simulink model "EiH_VFC_Renew_R2021b"  (R2021b)
settings: Solver=ode4  StartTime=0.0  StopTime=30  FixedStep=0.01  RelTol=1e-3
values from neighbouring files (symbols this model uses):
  denomi_threshold = 1e-8    (= 1e-08)    [param_EiH_VFC.m]
  Keo1 = Keo_Gain    (= 0.5)    [param_EiH_VFC.m]
  Keo2 = Keo_Gain    (= 0.5)    [param_EiH_VFC.m]
  Keo3 = Keo_Gain    (= 0.5)    [param_EiH_VFC.m]
  Keo4 = Keo_Gain    (= 0.5)    [param_EiH_VFC.m]
  Keo5 = Keo_Gain    (= 0.5)    [param_EiH_VFC.m]
  Keo6 = Keo_Gain    (= 0.5)    [param_EiH_VFC.m]
  Km1 = Km_gain    (= 0.1)    [param_EiH_VFC.m]
  Km2 = Km_gain    (= 0.1)    [param_EiH_VFC.m]
  Km3 = Km_gain    (= 0.1)    [param_EiH_VFC.m]
  Km4 = Km_gain    (= 0.1)    [param_EiH_VFC.m]
  Km5 = Km_gain    (= 0.1)    [param_EiH_VFC.m]
  Km6 = Km_gain    (= 0.1)    [param_EiH_VFC.m]
  pco_bar_init = pco_init + [0.15; 0.3; -0.1]    [param_EiH_VFC.m]
  pd = [1.0; 1.0; 0]    [param_EiH_VFC.m]
  Pinho_Para = [0; 0; 0; s_lambda_x; s_lambda_y]    [param_EiH_VFC.m]
  po = [xo1; yo1; zo1; xo2; yo2; zo2; xo3; yo3; zo3; xo4; yo4; zo4]    [param_EiH_VFC.m]
  pzeta_md = [pmd; zetamd]    [param_EiH_VFC.m]
  pzeta_wo_init = [pwo_init;zetawo_init]    [param_EiH_VFC.m]
  qwm_init = [0.0; 0.0; 0.0]    [param_EiH_VFC.m]
  R_threshold = 1e-8    (= 1e-08)    [param_EiH_VFC.m]
  Rco_bar_init = Rfromxi(zetaco_bar_init)    [param_EiH_VFC.m]
  theta_dz = 0.0    (= 0)    [param_EiH_VFC.m]
  zeta_threshold = 1e-8    (= 1e-08)    [param_EiH_VFC.m]
undefined symbols (not defined in the file or in its folder): Angle, Axis, magnitude, sx, sy
libraries: dspnetwork x2, dspmtrx3 x2, robotcorelib x1, vrlib x1
(part 2 of 4)

== system EiH_VFC_Renew_R2021b/make Ad(ge)/wedge ==
  "[3x1]" : Inport
  Product1 : Product  InputSameDT=on  SaturateOnIntegerOverflow=on  OutDataTypeStr=Inherit: Same as first input
  Product2 : Product  InputSameDT=on  SaturateOnIntegerOverflow=on  OutDataTypeStr=Inherit: Same as first input
  Product3 : Product  InputSameDT=on  SaturateOnIntegerOverflow=on  OutDataTypeStr=Inherit: Same as first input
  Sum : Sum  Inputs=+++  InputSameDT=on  SaturateOnIntegerOverflow=on  OutDataTypeStr=Inherit: Same as first input
  Xaxis : Constant  Value=[0 0 0;0 0 -1;0 1 0]  VectorParams1D=off
  Yaxis : Constant  Value=[0 0 1;0 0 0;-1 0 0]  VectorParams1D=off
  Zaxis : Constant  Value=[0 -1 0;1 0 0;0 0 0]  VectorParams1D=off
  x : Gain  Gain=[1 0 0]  Multiplication=Matrix(K*u)  SaturateOnIntegerOverflow=on  OutDataTypeStr=Inherit: Same as input  ParamDataTypeStr=Inherit: Same as input
  y : Gain  Gain=[0 1 0]  Multiplication=Matrix(K*u)  SaturateOnIntegerOverflow=on  OutDataTypeStr=Inherit: Same as input  ParamDataTypeStr=Inherit: Same as input
  z : Gain  Gain=[0 0 1]  Multiplication=Matrix(K*u)  SaturateOnIntegerOverflow=on  OutDataTypeStr=Inherit: Same as input  ParamDataTypeStr=Inherit: Same as input
  "[3x3]" : Outport  VectorParamsAs1DForOutWhenUnconnected=off
  wires:
  Sum/1 -> "[3x3]"/1
  Product1/1 -> Sum/3
  Product2/1 -> Sum/1
  Product3/1 -> Sum/2
  "[3x1]"/1 -> z/1, x/1, y/1
  y/1 -> Product3/1
  Yaxis/1 -> Product3/2
  x/1 -> Product2/1
  Xaxis/1 -> Product2/2
  z/1 -> Product1/1
  Zaxis/1 -> Product1/2

== system EiH_VFC_Renew_R2021b/make Rco pco/make p_zeta co ==
  "pco " : Inport
  Rco : Inport  Port=2
  Data pco : Subsystem
  Data zetaco : Subsystem
  Mux : Mux  Inputs=2
  make zeta_co : Subsystem
  pco WS : Subsystem
  "zeta_co WS " : Subsystem
  tag scope: p_zeta_co=global
  wires:
  "pco "/1 -> Data pco/1("pco "), pco WS/1(pco), Mux/1
  make zeta_co/1(zeta_co) -> "zeta_co WS "/1(zetaco), Data zetaco/1(zetaco), Mux/2
  Mux/1 -> [p_zeta_co]
  Rco/1 -> make zeta_co/1(Rco)

== system EiH_VFC_Renew_R2021b/make Rco pco/wedge ==
  "[3x1]" : Inport
  Product1 : Product  InputSameDT=on  SaturateOnIntegerOverflow=on  OutDataTypeStr=Inherit: Same as first input
  Product2 : Product  InputSameDT=on  SaturateOnIntegerOverflow=on  OutDataTypeStr=Inherit: Same as first input
  Product3 : Product  InputSameDT=on  SaturateOnIntegerOverflow=on  OutDataTypeStr=Inherit: Same as first input
  Sum : Sum  Inputs=+++  InputSameDT=on  SaturateOnIntegerOverflow=on  OutDataTypeStr=Inherit: Same as first input
  Xaxis : Constant  Value=[0 0 0;0 0 -1;0 1 0]  VectorParams1D=off
  Yaxis : Constant  Value=[0 0 1;0 0 0;-1 0 0]  VectorParams1D=off
  Zaxis : Constant  Value=[0 -1 0;1 0 0;0 0 0]  VectorParams1D=off
  x : Gain  Gain=[1 0 0]  Multiplication=Matrix(K*u)  SaturateOnIntegerOverflow=on  OutDataTypeStr=Inherit: Same as input  ParamDataTypeStr=Inherit: Same as input
  y : Gain  Gain=[0 1 0]  Multiplication=Matrix(K*u)  SaturateOnIntegerOverflow=on  OutDataTypeStr=Inherit: Same as input  ParamDataTypeStr=Inherit: Same as input
  z : Gain  Gain=[0 0 1]  Multiplication=Matrix(K*u)  SaturateOnIntegerOverflow=on  OutDataTypeStr=Inherit: Same as input  ParamDataTypeStr=Inherit: Same as input
  "[3x3]" : Outport  VectorParamsAs1DForOutWhenUnconnected=off
  wires:
  Sum/1 -> "[3x3]"/1
  Product1/1 -> Sum/3
  Product2/1 -> Sum/1
  Product3/1 -> Sum/2
  "[3x1]"/1 -> z/1, x/1, y/1
  y/1 -> Product3/1
  Yaxis/1 -> Product3/2
  x/1 -> Product2/1
  Xaxis/1 -> Product2/2
  z/1 -> Product1/1
  Zaxis/1 -> Product1/2

== system EiH_VFC_Renew_R2021b/make Rd pd/make_Rd ==
  zeta_d : Inport
  "3x1 -> 2norm" : Subsystem
  Constant : Constant
  I : Constant  Value=eye(3)  VectorParams1D=off
  I1 : Constant  Value=eye(3)  VectorParams1D=off
  Product : Product  InputSameDT=on  SaturateOnIntegerOverflow=on  OutDataTypeStr=Inherit: Same as first input
  Product1 : Product  InputSameDT=on  SaturateOnIntegerOverflow=on  OutDataTypeStr=Inherit: Same as first input
  Product2 : Product  Inputs=/  InputSameDT=on  SaturateOnIntegerOverflow=on  OutDataTypeStr=Inherit: Same as first input
  Product3 : Product  Multiplication=Matrix(*)  InputSameDT=on  SaturateOnIntegerOverflow=on  OutDataTypeStr=Inherit: Same as first input
  Product4 : Product  InputSameDT=on  SaturateOnIntegerOverflow=on  OutDataTypeStr=Inherit: Same as first input
  Sum : Sum  Inputs=+++  InputSameDT=on  SaturateOnIntegerOverflow=on  OutDataTypeStr=Inherit: Same as first input
  Sum1 : Sum  Inputs=|+-  InputSameDT=on  SaturateOnIntegerOverflow=on  OutDataTypeStr=Inherit: Same as first input
  Switch : Switch  Threshold=R_threshold  SaturateOnIntegerOverflow=on  InputSameDT=on
  cos(theta) : Trigonometry  Operator=cos
  sin(theta) : Trigonometry
  wedge : Subsystem
  zero check R_threshold : Subsystem
  Rd : Outport  VectorParamsAs1DForOutWhenUnconnected=off
  wires:
  Product3/1 -> Product1/1
  zeta_d/1 -> wedge/1("[3x1]"), "3x1 -> 2norm"/1(3x1)
  Product2/1 -> Product/2
  zero check R_threshold/1(Out1) -> cos(theta)/1, Switch/2, sin(theta)/1, Product2/1
  wedge/1("[3x3]") -> Product/1
  Product/1 -> Product3/2, Product3/1, Product4/1
  "3x1 -> 2norm"/1(2 norm) -> zero check R_threshold/1(In1)
  Switch/1 -> Rd/1
  I1/1 -> Switch/3
  Sum/1 -> Switch/1
  sin(theta)/1 -> Product4/2
  I/1 -> Sum/1
  Constant/1 -> Sum1/1
  cos(theta)/1 -> Sum1/2
  Sum1/1 -> Product1/2
  Product1/1 -> Sum/3
  Product4/1 -> Sum/2

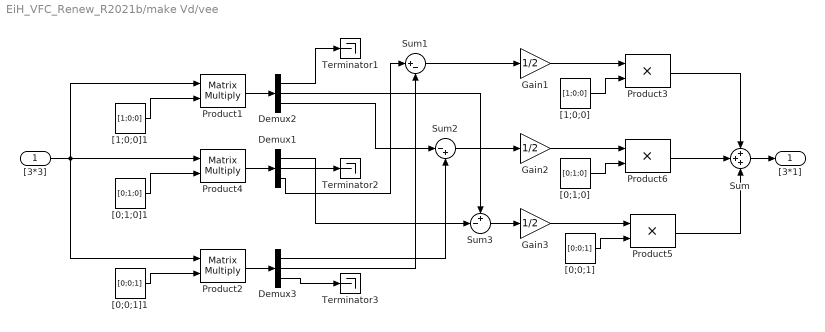
== system EiH_VFC_Renew_R2021b/make Vd/vee ==
  "[3*3]" : Inport
  Demux1 : Demux  Outputs=3
      settings: DisplayOption=none
  Demux2 : Demux  Outputs=3
      settings: DisplayOption=none
  Demux3 : Demux  Outputs=3
      settings: DisplayOption=none
  Gain1 : Gain  Gain=1/2  SaturateOnIntegerOverflow=on  OutDataTypeStr=Inherit: Same as input  ParamDataTypeStr=Inherit: Same as input
  Gain2 : Gain  Gain=1/2  SaturateOnIntegerOverflow=on  OutDataTypeStr=Inherit: Same as input  ParamDataTypeStr=Inherit: Same as input
  Gain3 : Gain  Gain=1/2  SaturateOnIntegerOverflow=on  OutDataTypeStr=Inherit: Same as input  ParamDataTypeStr=Inherit: Same as input
  Product1 : Product  Multiplication=Matrix(*)  InputSameDT=on  SaturateOnIntegerOverflow=on  OutDataTypeStr=Inherit: Same as first input
  Product2 : Product  Multiplication=Matrix(*)  InputSameDT=on  SaturateOnIntegerOverflow=on  OutDataTypeStr=Inherit: Same as first input
  Product3 : Product  InputSameDT=on  SaturateOnIntegerOverflow=on  OutDataTypeStr=Inherit: Same as first input
  Product4 : Product  Multiplication=Matrix(*)  InputSameDT=on  SaturateOnIntegerOverflow=on  OutDataTypeStr=Inherit: Same as first input
  Product5 : Product  InputSameDT=on  SaturateOnIntegerOverflow=on  OutDataTypeStr=Inherit: Same as first input
  Product6 : Product  InputSameDT=on  SaturateOnIntegerOverflow=on  OutDataTypeStr=Inherit: Same as first input
  Sum : Sum  Inputs=+++  InputSameDT=on  SaturateOnIntegerOverflow=on  OutDataTypeStr=Inherit: Same as first input
  Sum1 : Sum  Inputs=|+-  InputSameDT=on  SaturateOnIntegerOverflow=on  OutDataTypeStr=Inherit: Same as first input
  Sum2 : Sum  Inputs=|-+  InputSameDT=on  SaturateOnIntegerOverflow=on  OutDataTypeStr=Inherit: Same as first input
  Sum3 : Sum  Inputs=+-|  InputSameDT=on  SaturateOnIntegerOverflow=on  OutDataTypeStr=Inherit: Same as first input
  Terminator1 : Terminator
  Terminator2 : Terminator
  Terminator3 : Terminator
  "[0;0;1]" : Constant  Value=[0;0;1]  VectorParams1D=off
  "[0;0;1]1" : Constant  Value=[0;0;1]  VectorParams1D=off
  "[0;1;0]" : Constant  Value=[0;1;0]  VectorParams1D=off
  "[0;1;0]1" : Constant  Value=[0;1;0]  VectorParams1D=off
  "[1;0;0]" : Constant  Value=[1;0;0]  VectorParams1D=off
  "[1;0;0]1" : Constant  Value=[1;0;0]  VectorParams1D=off
  "[3*1]" : Outport  VectorParamsAs1DForOutWhenUnconnected=off
  wires:
  Demux1/1 -> Sum3/2
  Demux2/2 -> Sum3/1
  Sum3/1 -> Gain3/1
  Sum2/1 -> Gain2/1
  Demux2/3 -> Sum2/1
  Gain3/1 -> Product5/1
  Gain2/1 -> Product6/1
  Demux3/2 -> Sum1/2
  Gain1/1 -> Product3/1
  Sum1/1 -> Gain1/1
  Sum/1 -> "[3*1]"/1
  Product3/1 -> Sum/1
  Product5/1 -> Sum/3
  Product6/1 -> Sum/2
  "[0;0;1]"/1 -> Product5/2
  "[0;1;0]"/1 -> Product6/2
  "[1;0;0]"/1 -> Product3/2
  Demux3/1 -> Sum2/2
  Demux3/3 -> Terminator3/1
  Product2/1 -> Demux3/1
  "[0;0;1]1"/1 -> Product2/2
  Demux2/1 -> Terminator1/1
  Product1/1 -> Demux2/1
  "[1;0;0]1"/1 -> Product1/2
  Demux1/3 -> Sum1/1
  Demux1/2 -> Terminator2/1
  Product4/1 -> Demux1/1
  "[0;1;0]1"/1 -> Product4/2
  "[3*3]"/1 -> Product1/1, Product2/1, Product4/1

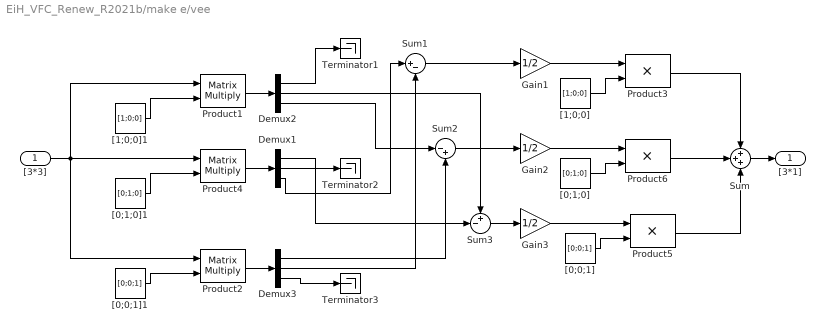
== system EiH_VFC_Renew_R2021b/make e/vee ==
  "[3*3]" : Inport
  Demux1 : Demux  Outputs=3
      settings: DisplayOption=none
  Demux2 : Demux  Outputs=3
      settings: DisplayOption=none
  Demux3 : Demux  Outputs=3
      settings: DisplayOption=none
  Gain1 : Gain  Gain=1/2  SaturateOnIntegerOverflow=on  OutDataTypeStr=Inherit: Same as input  ParamDataTypeStr=Inherit: Same as input
  Gain2 : Gain  Gain=1/2  SaturateOnIntegerOverflow=on  OutDataTypeStr=Inherit: Same as input  ParamDataTypeStr=Inherit: Same as input
  Gain3 : Gain  Gain=1/2  SaturateOnIntegerOverflow=on  OutDataTypeStr=Inherit: Same as input  ParamDataTypeStr=Inherit: Same as input
  Product1 : Product  Multiplication=Matrix(*)  InputSameDT=on  SaturateOnIntegerOverflow=on  OutDataTypeStr=Inherit: Same as first input
  Product2 : Product  Multiplication=Matrix(*)  InputSameDT=on  SaturateOnIntegerOverflow=on  OutDataTypeStr=Inherit: Same as first input
  Product3 : Product  InputSameDT=on  SaturateOnIntegerOverflow=on  OutDataTypeStr=Inherit: Same as first input
  Product4 : Product  Multiplication=Matrix(*)  InputSameDT=on  SaturateOnIntegerOverflow=on  OutDataTypeStr=Inherit: Same as first input
  Product5 : Product  InputSameDT=on  SaturateOnIntegerOverflow=on  OutDataTypeStr=Inherit: Same as first input
  Product6 : Product  InputSameDT=on  SaturateOnIntegerOverflow=on  OutDataTypeStr=Inherit: Same as first input
  Sum : Sum  Inputs=+++  InputSameDT=on  SaturateOnIntegerOverflow=on  OutDataTypeStr=Inherit: Same as first input
  Sum1 : Sum  Inputs=|+-  InputSameDT=on  SaturateOnIntegerOverflow=on  OutDataTypeStr=Inherit: Same as first input
  Sum2 : Sum  Inputs=|-+  InputSameDT=on  SaturateOnIntegerOverflow=on  OutDataTypeStr=Inherit: Same as first input
  Sum3 : Sum  Inputs=+-|  InputSameDT=on  SaturateOnIntegerOverflow=on  OutDataTypeStr=Inherit: Same as first input
  Terminator1 : Terminator
  Terminator2 : Terminator
  Terminator3 : Terminator
  "[0;0;1]" : Constant  Value=[0;0;1]  VectorParams1D=off
  "[0;0;1]1" : Constant  Value=[0;0;1]  VectorParams1D=off
  "[0;1;0]" : Constant  Value=[0;1;0]  VectorParams1D=off
  "[0;1;0]1" : Constant  Value=[0;1;0]  VectorParams1D=off
  "[1;0;0]" : Constant  Value=[1;0;0]  VectorParams1D=off
  "[1;0;0]1" : Constant  Value=[1;0;0]  VectorParams1D=off
  "[3*1]" : Outport  VectorParamsAs1DForOutWhenUnconnected=off
  wires:
  Demux1/1 -> Sum3/2
  Demux2/2 -> Sum3/1
  Sum3/1 -> Gain3/1
  Sum2/1 -> Gain2/1
  Demux2/3 -> Sum2/1
  Gain3/1 -> Product5/1
  Gain2/1 -> Product6/1
  Demux3/2 -> Sum1/2
  Gain1/1 -> Product3/1
  Sum1/1 -> Gain1/1
  Sum/1 -> "[3*1]"/1
  Product3/1 -> Sum/1
  Product5/1 -> Sum/3
  Product6/1 -> Sum/2
  "[0;0;1]"/1 -> Product5/2
  "[0;1;0]"/1 -> Product6/2
  "[1;0;0]"/1 -> Product3/2
  Demux3/1 -> Sum2/2
  Demux3/3 -> Terminator3/1
  Product2/1 -> Demux3/1
  "[0;0;1]1"/1 -> Product2/2
  Demux2/1 -> Terminator1/1
  Product1/1 -> Demux2/1
  "[1;0;0]1"/1 -> Product1/2
  Demux1/3 -> Sum1/1
  Demux1/2 -> Terminator2/1
  Product4/1 -> Demux1/1
  "[0;1;0]1"/1 -> Product4/2
  "[3*3]"/1 -> Product1/1, Product2/1, Product4/1

== system EiH_VFC_Renew_R2021b/make qe Re/Subsystem ==
  theta_dz : Inport
  Constant6 : Constant  Value=0
  Mux4 : Mux  Inputs=3
  make_Rd : Subsystem
  Rd : Outport
  wires:
  Constant6/1 -> Mux4/2, Mux4/1
  Mux4/1 -> make_Rd/1(zeta_d)
  theta_dz/1 -> Mux4/3
  make_Rd/1(Rd) -> Rd/1

== system EiH_VFC_Renew_R2021b/make zeta_wm/e_R(R) ==
  R : Inport
  sk(R) : Subsystem
  vee : Subsystem
  sk(R)^vee : Outport  VectorParamsAs1DForOutWhenUnconnected=off
  wires:
  sk(R)/1(sk(R)) -> vee/1("[3*3]")
  vee/1("[3*1]") -> sk(R)^vee/1
  R/1 -> sk(R)/1(R)

== system EiH_VFC_Renew_R2021b/make zeta_wm/make zeta ==
  sk(R)^vee : Inport
  "3x1 -> 2norm" : Subsystem
  Product : Product  InputSameDT=on  SaturateOnIntegerOverflow=on  OutDataTypeStr=Inherit: Same as first input
  Product1 : Product  Inputs=/  InputSameDT=on  SaturateOnIntegerOverflow=on  OutDataTypeStr=Inherit: Same as first input
  Product2 : Product  InputSameDT=on  SaturateOnIntegerOverflow=on  OutDataTypeStr=Inherit: Same as first input
  Switch : Switch  Threshold=zeta_threshold  SaturateOnIntegerOverflow=on  InputSameDT=on
  Trigonometric Function : Trigonometry  Operator=asin
  zero : Constant  Value=[0;0;0]  VectorParams1D=off
  zero check zeta_threshold : Subsystem
  zeta : Outport  VectorParamsAs1DForOutWhenUnconnected=off
  wires:
  Product2/1 -> Product/1
  Product1/1 -> Product2/2
  Trigonometric Function/1 -> Product2/1
  "3x1 -> 2norm"/1(2 norm) -> zero check zeta_threshold/1(In1)
  sk(R)^vee/1 -> Product/2, "3x1 -> 2norm"/1(3x1)
  zero check zeta_threshold/1(Out1) -> Trigonometric Function/1, Product1/1, Switch/2
  Switch/1 -> zeta/1
  Product/1 -> Switch/1
  zero/1 -> Switch/3

== system EiH_VFC_Renew_R2021b/pzeta_co_bar/  wedge   ==
  "[3x1]" : Inport
  Product1 : Product  InputSameDT=on  SaturateOnIntegerOverflow=on  OutDataTypeStr=Inherit: Same as first input
  Product2 : Product  InputSameDT=on  SaturateOnIntegerOverflow=on  OutDataTypeStr=Inherit: Same as first input
  Product3 : Product  InputSameDT=on  SaturateOnIntegerOverflow=on  OutDataTypeStr=Inherit: Same as first input
  Sum : Sum  Inputs=+++  InputSameDT=on  SaturateOnIntegerOverflow=on  OutDataTypeStr=Inherit: Same as first input
  Xaxis : Constant  Value=[0 0 0;0 0 -1;0 1 0]  VectorParams1D=off
  Yaxis : Constant  Value=[0 0 1;0 0 0;-1 0 0]  VectorParams1D=off
  Zaxis : Constant  Value=[0 -1 0;1 0 0;0 0 0]  VectorParams1D=off
  x : Gain  Gain=[1 0 0]  Multiplication=Matrix(K*u)  SaturateOnIntegerOverflow=on  OutDataTypeStr=Inherit: Same as input  ParamDataTypeStr=Inherit: Same as input
  y : Gain  Gain=[0 1 0]  Multiplication=Matrix(K*u)  SaturateOnIntegerOverflow=on  OutDataTypeStr=Inherit: Same as input  ParamDataTypeStr=Inherit: Same as input
  z : Gain  Gain=[0 0 1]  Multiplication=Matrix(K*u)  SaturateOnIntegerOverflow=on  OutDataTypeStr=Inherit: Same as input  ParamDataTypeStr=Inherit: Same as input
  "[3x3]" : Outport  VectorParamsAs1DForOutWhenUnconnected=off
  wires:
  Sum/1 -> "[3x3]"/1
  Product1/1 -> Sum/3
  Product2/1 -> Sum/1
  Product3/1 -> Sum/2
  "[3x1]"/1 -> z/1, x/1, y/1
  y/1 -> Product3/1
  Yaxis/1 -> Product3/2
  x/1 -> Product2/1
  Xaxis/1 -> Product2/2
  z/1 -> Product1/1
  Zaxis/1 -> Product1/2

== system EiH_VFC_Renew_R2021b/pzeta_co_bar/ wedge  ==
  "[3x1]" : Inport
  Product1 : Product  InputSameDT=on  SaturateOnIntegerOverflow=on  OutDataTypeStr=Inherit: Same as first input
  Product2 : Product  InputSameDT=on  SaturateOnIntegerOverflow=on  OutDataTypeStr=Inherit: Same as first input
  Product3 : Product  InputSameDT=on  SaturateOnIntegerOverflow=on  OutDataTypeStr=Inherit: Same as first input
  Sum : Sum  Inputs=+++  InputSameDT=on  SaturateOnIntegerOverflow=on  OutDataTypeStr=Inherit: Same as first input
  Xaxis : Constant  Value=[0 0 0;0 0 -1;0 1 0]  VectorParams1D=off
  Yaxis : Constant  Value=[0 0 1;0 0 0;-1 0 0]  VectorParams1D=off
  Zaxis : Constant  Value=[0 -1 0;1 0 0;0 0 0]  VectorParams1D=off
  x : Gain  Gain=[1 0 0]  Multiplication=Matrix(K*u)  SaturateOnIntegerOverflow=on  OutDataTypeStr=Inherit: Same as input  ParamDataTypeStr=Inherit: Same as input
  y : Gain  Gain=[0 1 0]  Multiplication=Matrix(K*u)  SaturateOnIntegerOverflow=on  OutDataTypeStr=Inherit: Same as input  ParamDataTypeStr=Inherit: Same as input
  z : Gain  Gain=[0 0 1]  Multiplication=Matrix(K*u)  SaturateOnIntegerOverflow=on  OutDataTypeStr=Inherit: Same as input  ParamDataTypeStr=Inherit: Same as input
  "[3x3]" : Outport  VectorParamsAs1DForOutWhenUnconnected=off
  wires:
  Zaxis/1 -> Product1/2
  z/1 -> Product1/1
  Xaxis/1 -> Product2/2
  x/1 -> Product2/1
  Yaxis/1 -> Product3/2
  y/1 -> Product3/1
  "[3x1]"/1 -> y/1, x/1, z/1
  Product3/1 -> Sum/2
  Product2/1 -> Sum/1
  Product1/1 -> Sum/3
  Sum/1 -> "[3x3]"/1

== system EiH_VFC_Renew_R2021b/pzeta_co_bar/wedge ==
  "[3x1]" : Inport
  Product1 : Product  InputSameDT=on  SaturateOnIntegerOverflow=on  OutDataTypeStr=Inherit: Same as first input
  Product2 : Product  InputSameDT=on  SaturateOnIntegerOverflow=on  OutDataTypeStr=Inherit: Same as first input
  Product3 : Product  InputSameDT=on  SaturateOnIntegerOverflow=on  OutDataTypeStr=Inherit: Same as first input
  Sum : Sum  Inputs=+++  InputSameDT=on  SaturateOnIntegerOverflow=on  OutDataTypeStr=Inherit: Same as first input
  Xaxis : Constant  Value=[0 0 0;0 0 -1;0 1 0]  VectorParams1D=off
  Yaxis : Constant  Value=[0 0 1;0 0 0;-1 0 0]  VectorParams1D=off
  Zaxis : Constant  Value=[0 -1 0;1 0 0;0 0 0]  VectorParams1D=off
  x : Gain  Gain=[1 0 0]  Multiplication=Matrix(K*u)  SaturateOnIntegerOverflow=on  OutDataTypeStr=Inherit: Same as input  ParamDataTypeStr=Inherit: Same as input
  y : Gain  Gain=[0 1 0]  Multiplication=Matrix(K*u)  SaturateOnIntegerOverflow=on  OutDataTypeStr=Inherit: Same as input  ParamDataTypeStr=Inherit: Same as input
  z : Gain  Gain=[0 0 1]  Multiplication=Matrix(K*u)  SaturateOnIntegerOverflow=on  OutDataTypeStr=Inherit: Same as input  ParamDataTypeStr=Inherit: Same as input
  "[3x3]" : Outport  VectorParamsAs1DForOutWhenUnconnected=off
  wires:
  Zaxis/1 -> Product1/2
  z/1 -> Product1/1
  Xaxis/1 -> Product2/2
  x/1 -> Product2/1
  Yaxis/1 -> Product3/2
  y/1 -> Product3/1
  "[3x1]"/1 -> y/1, x/1, z/1
  Product3/1 -> Sum/2
  Product2/1 -> Sum/1
  Product1/1 -> Sum/3
  Sum/1 -> "[3x3]"/1

== system EiH_VFC_Renew_R2021b/-Ka/Kcc/diag ==
  in[6*1] : Inport
  Constant1 : Constant  Value=[1 zeros(1,5);zeros(5,6)]  VectorParams1D=off
  Constant2 : Constant  Value=[zeros(1,6);0 1 zeros(1,4);zeros(4,6)]  VectorParams1D=off
  Constant4 : Constant  Value=[zeros(2,6);zeros(1,2) 1 zeros(1,3);zeros(3,6)]  VectorParams1D=off
  Constant5 : Constant  Value=[zeros(3,6);zeros(1,3) 1 zeros(1,2);zeros(2,6)]  VectorParams1D=off
  Constant6 : Constant  Value=[zeros(4,6);zeros(1,4) 1 zeros(1,1);zeros(1,6)]  VectorParams1D=off
  Constant7 : Constant  Value=[zeros(5,6);zeros(1,5) 1]  VectorParams1D=off
  Demux : Demux  Outputs=6
      settings: DisplayOption=none
  Product{,1..5} (6 alike) : Product  InputSameDT=on  SaturateOnIntegerOverflow=on  OutDataTypeStr=Inherit: Same as first input
  Sum : Sum  Inputs=++++++  InputSameDT=on  SaturateOnIntegerOverflow=on  OutDataTypeStr=Inherit: Same as first input
  diag : Outport  VectorParamsAs1DForOutWhenUnconnected=off
  wires:
  Demux/1 -> Product/1
  Constant1/1 -> Product/2
  Demux/2 -> Product1/1
  Constant2/1 -> Product1/2
  Demux/3 -> Product2/1
  Constant4/1 -> Product2/2
  Demux/4 -> Product3/1
  Constant5/1 -> Product3/2
  Constant6/1 -> Product4/2
  Demux/5 -> Product4/1
  Constant7/1 -> Product5/2
  Demux/6 -> Product5/1
  Product5/1 -> Sum/6
  Product4/1 -> Sum/5
  Product3/1 -> Sum/4
  Product2/1 -> Sum/3
  Product1/1 -> Sum/2
  Product/1 -> Sum/1
  in[6*1]/1 -> Demux/1
  Sum/1 -> diag/1

== system EiH_VFC_Renew_R2021b/-Keo/Keo/diag ==
  in[6*1] : Inport
  Constant1 : Constant  Value=[1 zeros(1,5);zeros(5,6)]  VectorParams1D=off
  Constant2 : Constant  Value=[zeros(1,6);0 1 zeros(1,4);zeros(4,6)]  VectorParams1D=off
  Constant4 : Constant  Value=[zeros(2,6);zeros(1,2) 1 zeros(1,3);zeros(3,6)]  VectorParams1D=off
  Constant5 : Constant  Value=[zeros(3,6);zeros(1,3) 1 zeros(1,2);zeros(2,6)]  VectorParams1D=off
  Constant6 : Constant  Value=[zeros(4,6);zeros(1,4) 1 zeros(1,1);zeros(1,6)]  VectorParams1D=off
  Constant7 : Constant  Value=[zeros(5,6);zeros(1,5) 1]  VectorParams1D=off
  Demux : Demux  Outputs=6
      settings: DisplayOption=none
  Product{,1..5} (6 alike) : Product  InputSameDT=on  SaturateOnIntegerOverflow=on  OutDataTypeStr=Inherit: Same as first input
  Sum : Sum  Inputs=++++++  InputSameDT=on  SaturateOnIntegerOverflow=on  OutDataTypeStr=Inherit: Same as first input
  diag : Outport  VectorParamsAs1DForOutWhenUnconnected=off
  wires:
  Demux/1 -> Product/1
  Constant1/1 -> Product/2
  Demux/2 -> Product1/1
  Constant2/1 -> Product1/2
  Demux/3 -> Product2/1
  Constant4/1 -> Product2/2
  Demux/4 -> Product3/1
  Constant5/1 -> Product3/2
  Constant6/1 -> Product4/2
  Demux/5 -> Product4/1
  Constant7/1 -> Product5/2
  Demux/6 -> Product5/1
  Product5/1 -> Sum/6
  Product4/1 -> Sum/5
  Product3/1 -> Sum/4
  Product2/1 -> Sum/3
  Product1/1 -> Sum/2
  Product/1 -> Sum/1
  in[6*1]/1 -> Demux/1
  Sum/1 -> diag/1

== system EiH_VFC_Renew_R2021b/-Km/Kcc/diag ==
  in[6*1] : Inport
  Constant1 : Constant  Value=[[1 0]; [0 0]]  VectorParams1D=off
  Constant2 : Constant  Value=[[0 0]; [0 1]]  VectorParams1D=off
  Demux : Demux  Outputs=2
      settings: DisplayOption=none
  Product : Product  InputSameDT=on  SaturateOnIntegerOverflow=on  OutDataTypeStr=Inherit: Same as first input
  Product1 : Product  InputSameDT=on  SaturateOnIntegerOverflow=on  OutDataTypeStr=Inherit: Same as first input
  Sum : Sum  InputSameDT=on  SaturateOnIntegerOverflow=on  OutDataTypeStr=Inherit: Same as first input
  diag : Outport  VectorParamsAs1DForOutWhenUnconnected=off
  wires:
  Demux/1 -> Product/1
  Constant1/1 -> Product/2
  Demux/2 -> Product1/1
  Constant2/1 -> Product1/2
  Product1/1 -> Sum/2
  Product/1 -> Sum/1
  in[6*1]/1 -> Demux/1
  Sum/1 -> diag/1

== system EiH_VFC_Renew_R2021b/Camera Model fco_bar/ fcq /fcq1 ==
  pc1 : Inport
  Pinho_Para : Inport  Port=2
  make fcqi : Subsystem
  fcq1 : Outport  VectorParamsAs1DForOutWhenUnconnected=off
  wires:
  Pinho_Para/1 -> make fcqi/2(Pinho_Para)
  make fcqi/1(fcqi) -> fcq1/1
  pc1/1 -> make fcqi/1(pci)

== system EiH_VFC_Renew_R2021b/Camera Model fco_bar/ fcq /fcq2 ==
  pc2 : Inport
  Pinho_Para : Inport  Port=2
  make fcqi : Subsystem
  fcq2 : Outport  VectorParamsAs1DForOutWhenUnconnected=off
  wires:
  Pinho_Para/1 -> make fcqi/2(Pinho_Para)
  make fcqi/1(fcqi) -> fcq2/1
  pc2/1 -> make fcqi/1(pci)

== system EiH_VFC_Renew_R2021b/Camera Model fco_bar/ fcq /fcq3 ==
  pc3 : Inport
  Pinho_Para : Inport  Port=2
  make fcqi : Subsystem
  fcq3 : Outport  VectorParamsAs1DForOutWhenUnconnected=off
  wires:
  Pinho_Para/1 -> make fcqi/2(Pinho_Para)
  make fcqi/1(fcqi) -> fcq3/1
  pc3/1 -> make fcqi/1(pci)

== system EiH_VFC_Renew_R2021b/Camera Model fco_bar/ fcq /fcq4 ==
  pc4 : Inport
  Pinho_Para : Inport  Port=2
  make fcqi : Subsystem
  fcq4 : Outport  VectorParamsAs1DForOutWhenUnconnected=off
  wires:
  Pinho_Para/1 -> make fcqi/2(Pinho_Para)
  make fcqi/1(fcqi) -> fcq4/1
  pc4/1 -> make fcqi/1(pci)

== system EiH_VFC_Renew_R2021b/Camera Model fco_bar/ fcq /pc1 ==
  pc : Inport
  Product4 : Product  Multiplication=Matrix(*)  InputSameDT=on  SaturateOnIntegerOverflow=on  OutDataTypeStr=Inherit: Same as first input
  eye(3) zero(3) zero(3) zero(3) : Constant  Value=[eye(3) zeros(3) zeros(3) zeros(3)]  VectorParams1D=off
  pc1 : Outport  VectorParamsAs1DForOutWhenUnconnected=off
  wires:
  pc/1 -> Product4/2
  Product4/1 -> pc1/1
  eye(3) zero(3) zero(3) zero(3)/1 -> Product4/1

== system EiH_VFC_Renew_R2021b/Camera Model fco_bar/ fcq /pc2 ==
  pc : Inport
  Product4 : Product  Multiplication=Matrix(*)  InputSameDT=on  SaturateOnIntegerOverflow=on  OutDataTypeStr=Inherit: Same as first input
  zero(3) eye(3) zero(3) zero(3) : Constant  Value=[zeros(3) eye(3) zeros(3) zeros(3)]  VectorParams1D=off
  pc2 : Outport  VectorParamsAs1DForOutWhenUnconnected=off
  wires:
  zero(3) eye(3) zero(3) zero(3)/1 -> Product4/1
  Product4/1 -> pc2/1
  pc/1 -> Product4/2

== system EiH_VFC_Renew_R2021b/Camera Model fco_bar/ fcq /pc3 ==
  pc : Inport
  Product4 : Product  Multiplication=Matrix(*)  InputSameDT=on  SaturateOnIntegerOverflow=on  OutDataTypeStr=Inherit: Same as first input
  zero(3) zero(3) eye(3) zero(3) : Constant  Value=[zeros(3) zeros(3) eye(3) zeros(3)]  VectorParams1D=off
  pc3 : Outport  VectorParamsAs1DForOutWhenUnconnected=off
  wires:
  pc/1 -> Product4/2
  Product4/1 -> pc3/1
  zero(3) zero(3) eye(3) zero(3)/1 -> Product4/1

== system EiH_VFC_Renew_R2021b/Camera Model fco_bar/ fcq /pc4 ==
  pc : Inport
  Product4 : Product  Multiplication=Matrix(*)  InputSameDT=on  SaturateOnIntegerOverflow=on  OutDataTypeStr=Inherit: Same as first input
  zero(3) zero(3) zero(3) eye(3) : Constant  Value=[zeros(3) zeros(3) zeros(3) eye(3)]  VectorParams1D=off
  pc4 : Outport  VectorParamsAs1DForOutWhenUnconnected=off
  wires:
  zero(3) zero(3) zero(3) eye(3)/1 -> Product4/1
  Product4/1 -> pc4/1
  pc/1 -> Product4/2

== system EiH_VFC_Renew_R2021b/Camera Model fco_bar/Feature Point Model/pc1 ==
  pcq : Inport
  Rcq : Inport  Port=2
  pq : Inport  Port=3
  Product1 : Product  Multiplication=Matrix(*)  InputSameDT=on  SaturateOnIntegerOverflow=on  OutDataTypeStr=Inherit: Same as first input
  Product4 : Product  Multiplication=Matrix(*)  InputSameDT=on  SaturateOnIntegerOverflow=on  OutDataTypeStr=Inherit: Same as first input
  Sum : Sum  Inputs=|++  InputSameDT=on  SaturateOnIntegerOverflow=on  OutDataTypeStr=Inherit: Same as first input
  eye(3) zero(3) zero(3) zero(3) : Constant  Value=[eye(3) zeros(3) zeros(3) zeros(3)]  VectorParams1D=off
  pc1 : Outport  VectorParamsAs1DForOutWhenUnconnected=off
  wires:
  pq/1 -> Product1/2
  Rcq/1 -> Product4/1
  Sum/1 -> pc1/1
  pcq/1 -> Sum/1
  Product1/1 -> Product4/2
  eye(3) zero(3) zero(3) zero(3)/1 -> Product1/1
  Product4/1 -> Sum/2

== system EiH_VFC_Renew_R2021b/Camera Model fco_bar/Feature Point Model/pc2 ==
  pcq : Inport
  Rcq : Inport  Port=2
  pq : Inport  Port=3
  Product1 : Product  Multiplication=Matrix(*)  InputSameDT=on  SaturateOnIntegerOverflow=on  OutDataTypeStr=Inherit: Same as first input
  Product4 : Product  Multiplication=Matrix(*)  InputSameDT=on  SaturateOnIntegerOverflow=on  OutDataTypeStr=Inherit: Same as first input
  Sum : Sum  Inputs=|++  InputSameDT=on  SaturateOnIntegerOverflow=on  OutDataTypeStr=Inherit: Same as first input
  zero(3) eye(3) zero(3) zero(3) : Constant  Value=[zeros(3) eye(3) zeros(3) zeros(3)]  VectorParams1D=off
  pc2 : Outport  VectorParamsAs1DForOutWhenUnconnected=off
  wires:
  Product4/1 -> Sum/2
  zero(3) eye(3) zero(3) zero(3)/1 -> Product1/1
  Product1/1 -> Product4/2
  pcq/1 -> Sum/1
  Sum/1 -> pc2/1
  Rcq/1 -> Product4/1
  pq/1 -> Product1/2

== system EiH_VFC_Renew_R2021b/Camera Model fco_bar/Feature Point Model/pc3 ==
  pcq : Inport
  Rcq : Inport  Port=2
  pq : Inport  Port=3
  Product1 : Product  Multiplication=Matrix(*)  InputSameDT=on  SaturateOnIntegerOverflow=on  OutDataTypeStr=Inherit: Same as first input
  Product4 : Product  Multiplication=Matrix(*)  InputSameDT=on  SaturateOnIntegerOverflow=on  OutDataTypeStr=Inherit: Same as first input
  Sum : Sum  Inputs=|++  InputSameDT=on  SaturateOnIntegerOverflow=on  OutDataTypeStr=Inherit: Same as first input
  zero(3) zero(3) eye(3) zero(3) : Constant  Value=[zeros(3) zeros(3) eye(3) zeros(3)]  VectorParams1D=off
  pc3 : Outport  VectorParamsAs1DForOutWhenUnconnected=off
  wires:
  pq/1 -> Product1/2
  Rcq/1 -> Product4/1
  Sum/1 -> pc3/1
  pcq/1 -> Sum/1
  Product1/1 -> Product4/2
  zero(3) zero(3) eye(3) zero(3)/1 -> Product1/1
  Product4/1 -> Sum/2

== system EiH_VFC_Renew_R2021b/Camera Model fco_bar/Feature Point Model/pc4 ==
  pcq : Inport
  Rcq : Inport  Port=2
  pq : Inport  Port=3
  Product1 : Product  Multiplication=Matrix(*)  InputSameDT=on  SaturateOnIntegerOverflow=on  OutDataTypeStr=Inherit: Same as first input
  Product4 : Product  Multiplication=Matrix(*)  InputSameDT=on  SaturateOnIntegerOverflow=on  OutDataTypeStr=Inherit: Same as first input
  Sum : Sum  Inputs=|++  InputSameDT=on  SaturateOnIntegerOverflow=on  OutDataTypeStr=Inherit: Same as first input
  zero(3) zero(3) zero(3) eye(3) : Constant  Value=[zeros(3) zeros(3) zeros(3) eye(3)]  VectorParams1D=off
  pc4 : Outport  VectorParamsAs1DForOutWhenUnconnected=off
  wires:
  Product4/1 -> Sum/2
  zero(3) zero(3) zero(3) eye(3)/1 -> Product1/1
  Product1/1 -> Product4/2
  pcq/1 -> Sum/1
  Sum/1 -> pc4/1
  Rcq/1 -> Product4/1
  pq/1 -> Product1/2

== system EiH_VFC_Renew_R2021b/Camera Model fco_bar/make p_zeta_co_bar/Data pco_bar ==
  pco_bar : Inport
  Demux : Demux  Outputs=3
      settings: DisplayOption=none
  pco_barx : Scope
  pco_bary : Scope
  pco_barz : Scope
  wires:
  Demux/3 -> pco_barz/1
  pco_bar/1 -> Demux/1
  Demux/2 -> pco_bary/1
  Demux/1 -> pco_barx/1

== system EiH_VFC_Renew_R2021b/Camera Model fco_bar/make p_zeta_co_bar/Data zetaco_bar ==
  zetaco_bar : Inport
  Demux : Demux  Outputs=3
      settings: DisplayOption=none
  zetaco_barx : Scope
  zetaco_bary : Scope
  zetaco_barz : Scope
  wires:
  Demux/3 -> zetaco_barz/1
  zetaco_bar/1 -> Demux/1
  Demux/2 -> zetaco_bary/1
  Demux/1 -> zetaco_barx/1

== system EiH_VFC_Renew_R2021b/Camera Model fco_bar/make p_zeta_co_bar/Rco_bar -> zeta_co_bar ==
  Rco_bar : Inport
  e_R(R) : Subsystem
  make zeta : Subsystem
  zeta_co_bar : Outport  VectorParamsAs1DForOutWhenUnconnected=off
  wires:
  e_R(R)/1(sk(R)^vee) -> make zeta/1(sk(R)^vee)
  Rco_bar/1 -> e_R(R)/1(R)
  make zeta/1(zeta) -> zeta_co_bar/1

== system EiH_VFC_Renew_R2021b/Camera Model fco_bar/make p_zeta_co_bar/Rco_bar WS ==
  Rco_bar : Inport
  To Workspace1 : ToWorkspace  VariableName=Rco_bar  SaveFormat=Structure  SampleTime=-1
  wires:
  Rco_bar/1 -> To Workspace1/1

== system EiH_VFC_Renew_R2021b/Camera Model fco_bar/make p_zeta_co_bar/pco_bar WS ==
  pco_bar : Inport
  Clock : Clock
  Demux4 : Demux  Outputs=3
      settings: DisplayOption=none
  Mux2 : Mux
  To Workspace1 : ToWorkspace  VariableName=pco_bar  SaveFormat=Structure  SampleTime=-1
  wires:
  pco_bar/1 -> Demux4/1
  Clock/1 -> Mux2/1
  Mux2/1 -> To Workspace1/1
  Demux4/3 -> Mux2/4
  Demux4/2 -> Mux2/3
  Demux4/1 -> Mux2/2

== system EiH_VFC_Renew_R2021b/Camera Model fco_bar/make p_zeta_co_bar/zetaco_bar WS ==
  zetaco_bar : Inport
  Clock : Clock
  Demux4 : Demux  Outputs=3
      settings: DisplayOption=none
  Mux2 : Mux
  To Workspace1 : ToWorkspace  VariableName=zetaco_bar  SaveFormat=Structure  SampleTime=-1
  wires:
  zetaco_bar/1 -> Demux4/1
  Clock/1 -> Mux2/1
  Mux2/1 -> To Workspace1/1
  Demux4/3 -> Mux2/4
  Demux4/2 -> Mux2/3
  Demux4/1 -> Mux2/2

== system EiH_VFC_Renew_R2021b/Image Jacobian fco/Image Jacobian/J1 ==
  pc1_bar : Inport
  Pinho_Para : Inport  Port=2
  Rcq_bar : Inport  Port=3
  pq1 : Inport  Port=4
  Ji_Left : Subsystem
  Ji_Right : Subsystem
  Product4 : Product  Multiplication=Matrix(*)  InputSameDT=on  SaturateOnIntegerOverflow=on  OutDataTypeStr=Inherit: Same as first input
  J1 : Outport  VectorParamsAs1DForOutWhenUnconnected=off
  wires:
  pc1_bar/1 -> Ji_Left/1(pci_bar)
  Ji_Left/1(Ji_Left) -> Product4/1
  Ji_Right/1(Ji_Right) -> Product4/2
  Pinho_Para/1 -> Ji_Left/2(Pinho_Para)
  Product4/1 -> J1/1
  Rcq_bar/1 -> Ji_Right/1(Rcq_bar)
  pq1/1 -> Ji_Right/2(pqi)

== system EiH_VFC_Renew_R2021b/Image Jacobian fco/Image Jacobian/J2 ==
  pc2_bar : Inport
  Pinho_Para : Inport  Port=2
  Rcq_bar : Inport  Port=3
  pq2 : Inport  Port=4
  Ji_Left : Subsystem
  Ji_Right : Subsystem
  Product4 : Product  Multiplication=Matrix(*)  InputSameDT=on  SaturateOnIntegerOverflow=on  OutDataTypeStr=Inherit: Same as first input
  J2 : Outport  VectorParamsAs1DForOutWhenUnconnected=off
  wires:
  pc2_bar/1 -> Ji_Left/1(pci_bar)
  Ji_Left/1(Ji_Left) -> Product4/1
  Ji_Right/1(Ji_Right) -> Product4/2
  Pinho_Para/1 -> Ji_Left/2(Pinho_Para)
  Product4/1 -> J2/1
  Rcq_bar/1 -> Ji_Right/1(Rcq_bar)
  pq2/1 -> Ji_Right/2(pqi)

== system EiH_VFC_Renew_R2021b/Image Jacobian fco/Image Jacobian/J3 ==
  pc3_bar : Inport
  Pinho_Para : Inport  Port=2
  Rcq_bar : Inport  Port=3
  pq3 : Inport  Port=4
  Ji_Left : Subsystem
  Ji_Right : Subsystem
  Product4 : Product  Multiplication=Matrix(*)  InputSameDT=on  SaturateOnIntegerOverflow=on  OutDataTypeStr=Inherit: Same as first input
  J3 : Outport  VectorParamsAs1DForOutWhenUnconnected=off
  wires:
  pc3_bar/1 -> Ji_Left/1(pci_bar)
  Ji_Left/1(Ji_Left) -> Product4/1
  Ji_Right/1(Ji_Right) -> Product4/2
  Pinho_Para/1 -> Ji_Left/2(Pinho_Para)
  Product4/1 -> J3/1
  Rcq_bar/1 -> Ji_Right/1(Rcq_bar)
  pq3/1 -> Ji_Right/2(pqi)

== system EiH_VFC_Renew_R2021b/Image Jacobian fco/Image Jacobian/J4 ==
  pc4_bar : Inport
  Pinho_Para : Inport  Port=2
  Rcq_bar : Inport  Port=3
  pq4 : Inport  Port=4
  Ji_Left : Subsystem
  Ji_Right : Subsystem
  Product4 : Product  Multiplication=Matrix(*)  InputSameDT=on  SaturateOnIntegerOverflow=on  OutDataTypeStr=Inherit: Same as first input
  J4 : Outport  VectorParamsAs1DForOutWhenUnconnected=off
  wires:
  pc4_bar/1 -> Ji_Left/1(pci_bar)
  Ji_Left/1(Ji_Left) -> Product4/1
  Ji_Right/1(Ji_Right) -> Product4/2
  Pinho_Para/1 -> Ji_Left/2(Pinho_Para)
  Product4/1 -> J4/1
  Rcq_bar/1 -> Ji_Right/1(Rcq_bar)
  pq4/1 -> Ji_Right/2(pqi)

== system EiH_VFC_Renew_R2021b/Image Jacobian fco/Image Jacobian/pc1 ==
  pc : Inport
  Product4 : Product  Multiplication=Matrix(*)  InputSameDT=on  SaturateOnIntegerOverflow=on  OutDataTypeStr=Inherit: Same as first input
  eye(3) zero(3) zero(3) zero(3) : Constant  Value=[eye(3) zeros(3) zeros(3) zeros(3)]  VectorParams1D=off
  pc1 : Outport  VectorParamsAs1DForOutWhenUnconnected=off
  wires:
  eye(3) zero(3) zero(3) zero(3)/1 -> Product4/1
  Product4/1 -> pc1/1
  pc/1 -> Product4/2

== system EiH_VFC_Renew_R2021b/Image Jacobian fco/Image Jacobian/pc2 ==
  pc : Inport
  Product4 : Product  Multiplication=Matrix(*)  InputSameDT=on  SaturateOnIntegerOverflow=on  OutDataTypeStr=Inherit: Same as first input
  zero(3) eye(3) zero(3) zero(3) : Constant  Value=[zeros(3) eye(3) zeros(3) zeros(3)]  VectorParams1D=off
  pc2 : Outport  VectorParamsAs1DForOutWhenUnconnected=off
  wires:
  zero(3) eye(3) zero(3) zero(3)/1 -> Product4/1
  Product4/1 -> pc2/1
  pc/1 -> Product4/2

== system EiH_VFC_Renew_R2021b/Image Jacobian fco/Image Jacobian/pc3 ==
  pc : Inport
  Product4 : Product  Multiplication=Matrix(*)  InputSameDT=on  SaturateOnIntegerOverflow=on  OutDataTypeStr=Inherit: Same as first input
  zero(3) zero(3) eye(3) zero(3) : Constant  Value=[zeros(3) zeros(3) eye(3) zeros(3)]  VectorParams1D=off
  pc3 : Outport  VectorParamsAs1DForOutWhenUnconnected=off
  wires:
  pc/1 -> Product4/2
  Product4/1 -> pc3/1
  zero(3) zero(3) eye(3) zero(3)/1 -> Product4/1

== system EiH_VFC_Renew_R2021b/Image Jacobian fco/Image Jacobian/pc4 ==
  pc : Inport
  Product4 : Product  Multiplication=Matrix(*)  InputSameDT=on  SaturateOnIntegerOverflow=on  OutDataTypeStr=Inherit: Same as first input
  zero(3) zero(3) zero(3) eye(3) : Constant  Value=[zeros(3) zeros(3) zeros(3) eye(3)]  VectorParams1D=off
  pc4 : Outport  VectorParamsAs1DForOutWhenUnconnected=off
  wires:
  zero(3) zero(3) zero(3) eye(3)/1 -> Product4/1
  Product4/1 -> pc4/1
  pc/1 -> Product4/2

== system EiH_VFC_Renew_R2021b/Image Jacobian fco/Image Jacobian/pq1 ==
  pq : Inport
  Product2 : Product  Multiplication=Matrix(*)  InputSameDT=on  SaturateOnIntegerOverflow=on  OutDataTypeStr=Inherit: Same as first input
  eye(3) zero(3) zero(3) zero(3) : Constant  Value=[eye(3) zeros(3) zeros(3) zeros(3)]  VectorParams1D=off
  pq1 : Outport  VectorParamsAs1DForOutWhenUnconnected=off
  wires:
  pq/1 -> Product2/2
  Product2/1 -> pq1/1
  eye(3) zero(3) zero(3) zero(3)/1 -> Product2/1

== system EiH_VFC_Renew_R2021b/Image Jacobian fco/Image Jacobian/pq2 ==
  pq : Inport
  Product2 : Product  Multiplication=Matrix(*)  InputSameDT=on  SaturateOnIntegerOverflow=on  OutDataTypeStr=Inherit: Same as first input
  zero(3) eye(3) zero(3) zero(3) : Constant  Value=[zeros(3) eye(3) zeros(3) zeros(3)]  VectorParams1D=off
  pq2 : Outport  VectorParamsAs1DForOutWhenUnconnected=off
  wires:
  zero(3) eye(3) zero(3) zero(3)/1 -> Product2/1
  Product2/1 -> pq2/1
  pq/1 -> Product2/2

== system EiH_VFC_Renew_R2021b/Image Jacobian fco/Image Jacobian/pq3 ==
  pq : Inport
  Product2 : Product  Multiplication=Matrix(*)  InputSameDT=on  SaturateOnIntegerOverflow=on  OutDataTypeStr=Inherit: Same as first input
  zero(3) zero(3) eye(3) zero(3) : Constant  Value=[zeros(3) zeros(3) eye(3) zeros(3)]  VectorParams1D=off
  pq3 : Outport  VectorParamsAs1DForOutWhenUnconnected=off
  wires:
  pq/1 -> Product2/2
  Product2/1 -> pq3/1
  zero(3) zero(3) eye(3) zero(3)/1 -> Product2/1

== system EiH_VFC_Renew_R2021b/Image Jacobian fco/Image Jacobian/pq4 ==
  pq : Inport
  Product2 : Product  Multiplication=Matrix(*)  InputSameDT=on  SaturateOnIntegerOverflow=on  OutDataTypeStr=Inherit: Same as first input
  zero(3) zero(3) zero(3) eye(3) : Constant  Value=[zeros(3) zeros(3) zeros(3) eye(3)]  VectorParams1D=off
  pq4 : Outport  VectorParamsAs1DForOutWhenUnconnected=off
  wires:
  zero(3) zero(3) zero(3) eye(3)/1 -> Product2/1
  Product2/1 -> pq4/1
  pq/1 -> Product2/2

== system EiH_VFC_Renew_R2021b/make Rco pco/make p_zeta co/Data pco ==
  "pco " : Inport
  Demux : Demux  Outputs=3
      settings: DisplayOption=none
  pco2_x : Scope
  pco2_y : Scope
  pco2_z : Scope
  wires:
  Demux/1 -> pco2_x/1
  Demux/2 -> pco2_y/1
  "pco "/1 -> Demux/1
  Demux/3 -> pco2_z/1

== system EiH_VFC_Renew_R2021b/make Rco pco/make p_zeta co/Data zetaco ==
  zetaco : Inport
  Demux : Demux  Outputs=3
      settings: DisplayOption=none
  zeta_co2_x : Scope
  zeta_co2_y : Scope
  zeta_co2_z : Scope
  wires:
  Demux/1 -> zeta_co2_x/1
  Demux/2 -> zeta_co2_y/1
  zetaco/1 -> Demux/1
  Demux/3 -> zeta_co2_z/1

== system EiH_VFC_Renew_R2021b/make Rco pco/make p_zeta co/make zeta_co ==
  Rco : Inport
  e_R(R) : Subsystem
  make zeta : Subsystem
  zeta_co : Outport  VectorParamsAs1DForOutWhenUnconnected=off
  wires:
  e_R(R)/1(sk(R)^vee) -> make zeta/1(sk(R)^vee)
  Rco/1 -> e_R(R)/1(R)
  make zeta/1(zeta) -> zeta_co/1

== system EiH_VFC_Renew_R2021b/make Rco pco/make p_zeta co/pco WS ==
  pco : Inport
  Clock : Clock
  Demux4 : Demux  Outputs=3
      settings: DisplayOption=none
  Mux2 : Mux
  To Workspace1 : ToWorkspace  VariableName=pco2  SaveFormat=Structure  SampleTime=-1
  wires:
  Demux4/1 -> Mux2/2
  Demux4/2 -> Mux2/3
  Demux4/3 -> Mux2/4
  Mux2/1 -> To Workspace1/1
  Clock/1 -> Mux2/1
  pco/1 -> Demux4/1

== system EiH_VFC_Renew_R2021b/make Rco pco/make p_zeta co/zeta_co WS  ==
  zetaco : Inport
  Clock : Clock
  Demux4 : Demux  Outputs=3
      settings: DisplayOption=none
  Mux2 : Mux
  To Workspace1 : ToWorkspace  VariableName=zetaco2  SaveFormat=Structure  SampleTime=-1
  wires:
  Demux4/1 -> Mux2/2
  Demux4/2 -> Mux2/3
  Demux4/3 -> Mux2/4
  Mux2/1 -> To Workspace1/1
  Clock/1 -> Mux2/1
  zetaco/1 -> Demux4/1

== system EiH_VFC_Renew_R2021b/make Rd pd/make_Rd/3x1 -> 2norm ==
  3x1 : Inport
  Demux : Demux  Outputs=3
      settings: DisplayOption=none
  Math Function : Math  Operator=magnitude^2  SignedPower=on  SaturateOnIntegerOverflow=on
  Math Function1 : Math  Operator=sqrt  SignedPower=on  SaturateOnIntegerOverflow=on
  Sum : Sum  Inputs=+++  InputSameDT=on  SaturateOnIntegerOverflow=on  OutDataTypeStr=Inherit: Same as first input
  2 norm : Outport  VectorParamsAs1DForOutWhenUnconnected=off
  wires:
  Math Function/1 -> Demux/1
  Demux/3 -> Sum/3
  Demux/2 -> Sum/2
  Demux/1 -> Sum/1
  Sum/1 -> Math Function1/1
  Math Function1/1 -> 2 norm/1
  3x1/1 -> Math Function/1

== system EiH_VFC_Renew_R2021b/make Rd pd/make_Rd/wedge ==
  "[3x1]" : Inport
  Product1 : Product  InputSameDT=on  SaturateOnIntegerOverflow=on  OutDataTypeStr=Inherit: Same as first input
  Product2 : Product  InputSameDT=on  SaturateOnIntegerOverflow=on  OutDataTypeStr=Inherit: Same as first input
  Product3 : Product  InputSameDT=on  SaturateOnIntegerOverflow=on  OutDataTypeStr=Inherit: Same as first input
  Sum : Sum  Inputs=+++  InputSameDT=on  SaturateOnIntegerOverflow=on  OutDataTypeStr=Inherit: Same as first input
  Xaxis : Constant  Value=[0 0 0;0 0 -1;0 1 0]  VectorParams1D=off
  Yaxis : Constant  Value=[0 0 1;0 0 0;-1 0 0]  VectorParams1D=off
  Zaxis : Constant  Value=[0 -1 0;1 0 0;0 0 0]  VectorParams1D=off
  x : Gain  Gain=[1 0 0]  Multiplication=Matrix(K*u)  SaturateOnIntegerOverflow=on  OutDataTypeStr=Inherit: Same as input  ParamDataTypeStr=Inherit: Same as input
  y : Gain  Gain=[0 1 0]  Multiplication=Matrix(K*u)  SaturateOnIntegerOverflow=on  OutDataTypeStr=Inherit: Same as input  ParamDataTypeStr=Inherit: Same as input
  z : Gain  Gain=[0 0 1]  Multiplication=Matrix(K*u)  SaturateOnIntegerOverflow=on  OutDataTypeStr=Inherit: Same as input  ParamDataTypeStr=Inherit: Same as input
  "[3x3]" : Outport  VectorParamsAs1DForOutWhenUnconnected=off
  wires:
  Sum/1 -> "[3x3]"/1
  Product1/1 -> Sum/3
  Product2/1 -> Sum/1
  Product3/1 -> Sum/2
  "[3x1]"/1 -> z/1, x/1, y/1
  y/1 -> Product3/1
  Yaxis/1 -> Product3/2
  x/1 -> Product2/1
  Xaxis/1 -> Product2/2
  z/1 -> Product1/1
  Zaxis/1 -> Product1/2

== system EiH_VFC_Renew_R2021b/make Rd pd/make_Rd/zero check R_threshold ==
  In1 : Inport
  Switch : Switch  Threshold=R_threshold  SaturateOnIntegerOverflow=on  InputSameDT=on
  norm_xi : Constant  Value=R_threshold  VectorParams1D=off
  Out1 : Outport  VectorParamsAs1DForOutWhenUnconnected=off
  wires:
  Switch/1 -> Out1/1
  In1/1 -> Switch/2, Switch/1
  norm_xi/1 -> Switch/3

== system EiH_VFC_Renew_R2021b/make qe Re/Subsystem/make_Rd ==
  zeta_d : Inport
  "3x1 -> 2norm" : Subsystem
  Constant : Constant
  I : Constant  Value=eye(3)  VectorParams1D=off
  I1 : Constant  Value=eye(3)  VectorParams1D=off
  Product : Product  InputSameDT=on  SaturateOnIntegerOverflow=on  OutDataTypeStr=Inherit: Same as first input
  Product1 : Product  InputSameDT=on  SaturateOnIntegerOverflow=on  OutDataTypeStr=Inherit: Same as first input
  Product2 : Product  Inputs=/  InputSameDT=on  SaturateOnIntegerOverflow=on  OutDataTypeStr=Inherit: Same as first input
  Product3 : Product  Multiplication=Matrix(*)  InputSameDT=on  SaturateOnIntegerOverflow=on  OutDataTypeStr=Inherit: Same as first input
  Product4 : Product  InputSameDT=on  SaturateOnIntegerOverflow=on  OutDataTypeStr=Inherit: Same as first input
  Sum : Sum  Inputs=+++  InputSameDT=on  SaturateOnIntegerOverflow=on  OutDataTypeStr=Inherit: Same as first input
  Sum1 : Sum  Inputs=|+-  InputSameDT=on  SaturateOnIntegerOverflow=on  OutDataTypeStr=Inherit: Same as first input
  Switch : Switch  Threshold=R_threshold  SaturateOnIntegerOverflow=on  InputSameDT=on
  cos(theta) : Trigonometry  Operator=cos
  sin(theta) : Trigonometry
  wedge : Subsystem
  zero check R_threshold : Subsystem
  Rd : Outport  VectorParamsAs1DForOutWhenUnconnected=off
  wires:
  Product3/1 -> Product1/1
  zeta_d/1 -> wedge/1("[3x1]"), "3x1 -> 2norm"/1(3x1)
  Product2/1 -> Product/2
  zero check R_threshold/1(Out1) -> cos(theta)/1, Switch/2, sin(theta)/1, Product2/1
  wedge/1("[3x3]") -> Product/1
  Product/1 -> Product3/2, Product3/1, Product4/1
  "3x1 -> 2norm"/1(2 norm) -> zero check R_threshold/1(In1)
  Switch/1 -> Rd/1
  I1/1 -> Switch/3
  Sum/1 -> Switch/1
  sin(theta)/1 -> Product4/2
  I/1 -> Sum/1
  Constant/1 -> Sum1/1
  cos(theta)/1 -> Sum1/2
  Sum1/1 -> Product1/2
  Product1/1 -> Sum/3
  Product4/1 -> Sum/2

== system EiH_VFC_Renew_R2021b/make zeta_wm/e_R(R)/sk(R) ==
  R : Inport
  Gain : Gain  Gain=1/2  SaturateOnIntegerOverflow=on  OutDataTypeStr=Inherit: Same as input  ParamDataTypeStr=Inherit: Same as input
  Math Function2 : Math  Operator=transpose  SignedPower=on  SaturateOnIntegerOverflow=on
  Sum : Sum  Inputs=|+-  InputSameDT=on  SaturateOnIntegerOverflow=on  OutDataTypeStr=Inherit: Same as first input
  sk(R) : Outport  VectorParamsAs1DForOutWhenUnconnected=off
  wires:
  R/1 -> Math Function2/1, Sum/1
  Math Function2/1 -> Sum/2
  Sum/1 -> Gain/1
  Gain/1 -> sk(R)/1

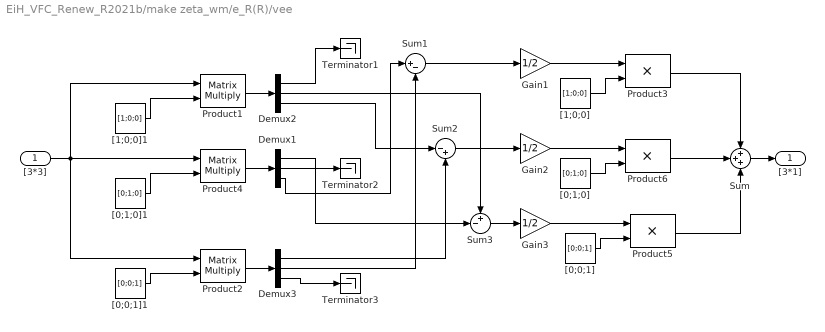
== system EiH_VFC_Renew_R2021b/make zeta_wm/e_R(R)/vee ==
  "[3*3]" : Inport
  Demux1 : Demux  Outputs=3
      settings: DisplayOption=none
  Demux2 : Demux  Outputs=3
      settings: DisplayOption=none
  Demux3 : Demux  Outputs=3
      settings: DisplayOption=none
  Gain1 : Gain  Gain=1/2  SaturateOnIntegerOverflow=on  OutDataTypeStr=Inherit: Same as input  ParamDataTypeStr=Inherit: Same as input
  Gain2 : Gain  Gain=1/2  SaturateOnIntegerOverflow=on  OutDataTypeStr=Inherit: Same as input  ParamDataTypeStr=Inherit: Same as input
  Gain3 : Gain  Gain=1/2  SaturateOnIntegerOverflow=on  OutDataTypeStr=Inherit: Same as input  ParamDataTypeStr=Inherit: Same as input
  Product1 : Product  Multiplication=Matrix(*)  InputSameDT=on  SaturateOnIntegerOverflow=on  OutDataTypeStr=Inherit: Same as first input
  Product2 : Product  Multiplication=Matrix(*)  InputSameDT=on  SaturateOnIntegerOverflow=on  OutDataTypeStr=Inherit: Same as first input
  Product3 : Product  InputSameDT=on  SaturateOnIntegerOverflow=on  OutDataTypeStr=Inherit: Same as first input
  Product4 : Product  Multiplication=Matrix(*)  InputSameDT=on  SaturateOnIntegerOverflow=on  OutDataTypeStr=Inherit: Same as first input
  Product5 : Product  InputSameDT=on  SaturateOnIntegerOverflow=on  OutDataTypeStr=Inherit: Same as first input
  Product6 : Product  InputSameDT=on  SaturateOnIntegerOverflow=on  OutDataTypeStr=Inherit: Same as first input
  Sum : Sum  Inputs=+++  InputSameDT=on  SaturateOnIntegerOverflow=on  OutDataTypeStr=Inherit: Same as first input
  Sum1 : Sum  Inputs=|+-  InputSameDT=on  SaturateOnIntegerOverflow=on  OutDataTypeStr=Inherit: Same as first input
  Sum2 : Sum  Inputs=|-+  InputSameDT=on  SaturateOnIntegerOverflow=on  OutDataTypeStr=Inherit: Same as first input
  Sum3 : Sum  Inputs=+-|  InputSameDT=on  SaturateOnIntegerOverflow=on  OutDataTypeStr=Inherit: Same as first input
  Terminator1 : Terminator
  Terminator2 : Terminator
  Terminator3 : Terminator
  "[0;0;1]" : Constant  Value=[0;0;1]  VectorParams1D=off
  "[0;0;1]1" : Constant  Value=[0;0;1]  VectorParams1D=off
  "[0;1;0]" : Constant  Value=[0;1;0]  VectorParams1D=off
  "[0;1;0]1" : Constant  Value=[0;1;0]  VectorParams1D=off
  "[1;0;0]" : Constant  Value=[1;0;0]  VectorParams1D=off
  "[1;0;0]1" : Constant  Value=[1;0;0]  VectorParams1D=off
  "[3*1]" : Outport  VectorParamsAs1DForOutWhenUnconnected=off
  wires:
  "[3*3]"/1 -> Product2/1, Product1/1, Product4/1
  "[0;1;0]1"/1 -> Product4/2
  Product4/1 -> Demux1/1
  Demux1/2 -> Terminator2/1
  Demux1/3 -> Sum1/1
  "[1;0;0]1"/1 -> Product1/2
  Product1/1 -> Demux2/1
  Demux2/1 -> Terminator1/1
  "[0;0;1]1"/1 -> Product2/2
  Product2/1 -> Demux3/1
  Demux3/3 -> Terminator3/1
  Demux3/1 -> Sum2/2
  "[1;0;0]"/1 -> Product3/2
  "[0;1;0]"/1 -> Product6/2
  "[0;0;1]"/1 -> Product5/2
  Product6/1 -> Sum/2
  Product5/1 -> Sum/3
  Product3/1 -> Sum/1
  Sum/1 -> "[3*1]"/1
  Sum1/1 -> Gain1/1
  Gain1/1 -> Product3/1
  Demux3/2 -> Sum1/2
  Gain2/1 -> Product6/1
  Gain3/1 -> Product5/1
  Demux2/3 -> Sum2/1
  Sum2/1 -> Gain2/1
  Sum3/1 -> Gain3/1
  Demux2/2 -> Sum3/1
  Demux1/1 -> Sum3/2

== system EiH_VFC_Renew_R2021b/make zeta_wm/make zeta/3x1 -> 2norm ==
  3x1 : Inport
  Demux : Demux  Outputs=3
      settings: DisplayOption=none
  Math Function : Math  Operator=magnitude^2  SignedPower=on  SaturateOnIntegerOverflow=on
  Math Function1 : Math  Operator=sqrt  SignedPower=on  SaturateOnIntegerOverflow=on
  Sum : Sum  Inputs=+++  InputSameDT=on  SaturateOnIntegerOverflow=on  OutDataTypeStr=Inherit: Same as first input
  2 norm : Outport  VectorParamsAs1DForOutWhenUnconnected=off
  wires:
  Math Function/1 -> Demux/1
  Demux/3 -> Sum/3
  Demux/2 -> Sum/2
  Demux/1 -> Sum/1
  Sum/1 -> Math Function1/1
  Math Function1/1 -> 2 norm/1
  3x1/1 -> Math Function/1

== system EiH_VFC_Renew_R2021b/make zeta_wm/make zeta/zero check zeta_threshold ==
  In1 : Inport
  Switch : Switch  Threshold=zeta_threshold  SaturateOnIntegerOverflow=on  InputSameDT=on
  norm_eR : Constant  Value=zeta_threshold  VectorParams1D=off
  Out1 : Outport  VectorParamsAs1DForOutWhenUnconnected=off
  wires:
  norm_eR/1 -> Switch/3
  In1/1 -> Switch/1, Switch/2
  Switch/1 -> Out1/1
